simulink library "svm_lib"  (Simulink 8.6)
settings: Solver=VariableStepAuto  StartTime=0.0  StopTime=10.0  RelTol=1e-3
values from neighbouring files (symbols this model uses):
  My_3D = ([eye(6) -eye(6)])    [svm_buildLinearControllers.m]    (also in svm_setup.m = [-eye(6) eye(6)])
  turbulence2loadfactors = blkdiag(T_w2nx, T_w2nz)    [svm_buildLinearControllers.m]
  uavsim = loaded.uavsim    [svm_sandbox.m]
undefined symbols (not defined in the file or in its folder): dt, F, fflib_delay_c2d, Light, mask_p0_NED, mask_v0_NED, MIL, postracking, svm, uavsimblockset_cartesianToAngle
libraries: svm_lib x9, simulink_extras x8, aerolibtransform2 x3, formationFlyingBlockset x2, uavsimBlockset_Cularis_Aerandpropulsion x1, uavsimBlockset_ElectricPropulsion x1, aerolibwind2 x1, aerolibgravity2 x1, uavsimBlockset_VectorNorm x1, uavsimBlockset_UAV3DInterface x1
(part 3 of 3)

== system svm_lib/Standard Vehicle Model/Inner loop dynamics/Second order models ==
  u : Inport
  Bus Selector : BusSelector  OutputSignals=n
  Bus Object Bus Creator : BusCreator  Inputs=2  OutDataTypeStr=Bus: svm_bus_xi  mask(BUS OBJECT Bus Creator){busType=Bus: svm_bus_xi}
      mask prompts: busType "Bus Type"
      mask help:
      | Provides users the cabability to painlessly, instantly customize bus creators of output data type 'Bus:' by selecting the bus object type from a drop down menu dynamically populated by bus objects in the workspace.
      |
      | After pressing the "Apply Selection" button signal lines into the creator are populated and named with the elements in the chosen bus saving the user from having to recall and fill out signal line names.
      |
      | NOTE that when copying a Bus Object Bus Creator from your locked Library the link to the Library is automatically broken. This saves the user from having to Unlock Links To Library (From the Library menu.), Disable Link and finally Break Link (Both from the Model menu.) for every placed instance of the block.
      settings: AttributesFormatString=%<OutDataTypeStr>  CopyFcn=set_param(gcb, 'LinkStatus', 'none')
      mask TypeOptions busType: Bus: AHRS | Bus: Acceleration | Bus: Aero | Bus: Airdata | Bus: Airframe | Bus: Attitude | Bus: CMD | Bus: CMD_quadrotor | Bus: ControlInfoBus | Bus: Enginedata | Bus: Environment | Bus: FlightGearData | Bus: GCSUpstream | Bus: GNSSL1 | Bus: GNSSRTK | Bus: GPS | Bus: IMU | Bus: Kinematics | Bus: LandinggearInput | Bus: MotionTracker | Bus: Position | Bus: Radiodistance | Bus: RotationalAcceleration | Bus: RotationalVelocity | Bus: SensorBus | Bus: StateBus | Bus: Velocity | Bus: WindAngles | Bus: iUAScom | Bus: svm_bus_d_exo | Bus: svm_bus_u_scaled | Bus: svm_bus_x | Bus: svm_bus_xi
      mask Callback busType:
      | % Using variable names terminated with "_BOBC" to lessen the chances of
      | % collisions with existing workspace variables.
      | 
      | % Get the current block handle and mask handle.
      | handleCreator_BOBC = gcbh;
      | maskObj_BOBC       = Simulink.Mask.get(gcb);
      | 
      | % Get a list of variables in the workspace in order to search for the '1x1
      | % Bus' types.
      | wsVars_BOBC = whos;
      | 
      | % Reset the 'TypeOptions' bus list in case some '1x1 Bus' types have been
      | % deleted from or added to the workspace.
      | maskObj_BOBC.Parameters.TypeOptions = {'<empty>'};
      | 
      | % Reset the bus count.
      | busCount_BOBC = 0;
      | 
      | for index_BOBC = 1:length(wsVars_BOBC)
      | 
      |    % If the variable is a bus object...
      |    if strcmp(wsVars_BOBC(index_BOBC).class, 'Simulink.Bus')
      | 
      |       busCount_BOBC = busCount_BOBC + 1;
      | 
      |       % ... add it to the TypeOptions of the mask.
      |       maskObj_BOBC.Parameters.TypeOptions(busCount_BOBC) = ...
      |                                                            ...
      |                                  {['Bus: ', wsVars_BOBC(index_BOBC).name]};
      |    end
      | end
      | 
      | if busCount_BOBC == 0
      | 
      |    % If there are NO bus objects in the workspace then provide a warning
      |    % popup...
      |    warndlg('There are currently no bus objects in the workspace - you have no use for this block. Use a normal Bus Creator instead.')
      | 
      |    % ... and do nothing.
      | elseif ~strcmp(get_param(handleCreator_BOBC, 'OutDataTypeStr'), 'Inherit: auto')
      | 
      |    % If the currently selected bus data type ('OutDataTypeStr') is not
      |    % 'Inherit: auto' (i.e., if we are reopening the mask.) then get the
      |    % current 'OutDataTypeStr' and 'maskVal.' ('maskVal' is the selected
      |    % 'TypeOptions' list member.)
      |    outDatStr_BOBC = get_param(handleCreator_BOBC, 'OutDataTypeStr');
      |    maskVal_BOBC   = get_param(handleCreator_BOBC, 'MaskValues');
      | 
      |    if ~strcmp(outDatStr_BOBC, maskVal_BOBC{1})
      | 
      |       % Upon re-opening the mask if the default 'TypeOptions' list member
      |       % (The first one.) contained in 'maskVal' does not match the
      |       % currently selected bus data type ('OutDataTypeStr') then set the
      |       % 'TypeOptions' list member to the selected bus data type. (Cuts down
      |       % on confusion to have the displayed list member match the selected
      |       % bus data type rather than the first entry.)
      |       set_param(handleCreator_BOBC, 'MaskValues', {outDatStr_BOBC});
      |    end
      | end
      | 
      | % Clean up the workspace.
      | clear  handleCreator_BOBC  maskObj_BOBC     wsVars_BOBC ...
      |             busCount_BOBC    index_BOBC  outDatStr_BOBC ...
      |              maskVal_BOBC
      mask DialogControl applyMOCBSelection Prompt: Apply Selection
      mask DialogControl applyMOCBSelection Callback:
      | % Using variable names terminated with "_BOBC" to lessen the chances of
      | % collisions with existing workspace variables.
      | 
      | % Get the current block, current block handle and mask handle.
      | currentBlock_BOBC  = gcb;
      | handleCreator_BOBC = gcbh;
      | 
      | % Get the desired bus type...
      | desiredBusType_BOBC = get_param(handleCreator_BOBC, 'busType');
      | 
      | % ... and set the 'OutDataTypeStr' to it.
      | set_param(handleCreator_BOBC, 'OutDataTypeStr', desiredBusType_BOBC);
      | 
      | %% First delete any existing lines on the port.
      | % Get the line handles.
      | lh_BOBC = get_param(handleCreator_BOBC, 'LineHandles');
      | 
      | % If any lines exist (Non- -1 line handles.), delete them and start over.
      | if max(lh_BOBC.Inport > 0)
      | 
      |    for index_BOBC = 1:length(lh_BOBC.Inport)
      | 
      |       if lh_BOBC.Inport(index_BOBC) > 0
      | 
      |          delete_line(lh_BOBC.Inport(index_BOBC))
      |       end
      |    end
      | end
      | 
      | %% Then work on adding new lines.
      | 
      | % Get the block path for 'add_line' function.
      | blockPath_BOBC = get_param(handleCreator_BOBC, 'Parent');
      | 
      | % Get the newly selected bus type ('OutDataTypeStr')...
      | mocbBusType_BOBC = get_param(currentBlock_BOBC, 'OutDataTypeStr');
      | 
      | % ... and parse off "Bus: " so the string of the desired bus contained in
      | % 'OutDataTypeStr' matches the raw workspace bus names.
      | mocbBusType_BOBC = mocbBusType_BOBC(6:end);
      | 
      | % Then evaluate the string containing the workspace bus name which will
      | % load the desired bus parameters.
      | busParams_BOBC = eval(mocbBusType_BOBC);
      | 
      | % From the parameters grab the number of lines to add.
      | numLines_BOBC = length(busParams_BOBC.Elements);
      | 
      | % Set the number of inputs of the masked bus creator to the number of lines
      | % to add.
      | set_param(handleCreator_BOBC, 'Inputs', num2str(numLines_BOBC));
      | 
      | % Get (Inputs.) port handles so we can grab the positions of them.
      | ph_BOBC = get_param(handleCreator_BOBC, 'PortHandles');
      | 
      | for index_BOBC = 1:numLines_BOBC
      | 
      |    % Get the position of input port number 'index_BOBC'.
      |    portPos_BOBC = get_param(ph_BOBC.Inport(index_BOBC), 'Position');
      | 
      |    % Add a line from 50 pixels left of the port position to the port
      |    % position. (This must be done because it's the lines that get named,
      |    % not the port positions.)
      |    portLine_BOBC = add_line(blockPath_BOBC, [portPos_BOBC - [50 0]; portPos_BOBC]);
      | 
      |    % Rename the new line to the bus 'index_BOBC-st/nd/rd/th' element name.
      |    set_param(portLine_BOBC, 'Name', busParams_BOBC.Elements(index_BOBC).Name)
      | end
      | 
      | %% Cleanup the workspace.
      | clear    currentBlock_BOBC  handleCreator_BOBC      index_BOBC ...
      |        desiredBusType_BOBC             lh_BOBC  blockPath_BOBC ...
      |           mocbBusType_BOBC      busParams_BOBC   numLines_BOBC ...
      |                    ph_BOBC        portPos_BOBC   portLine_BOBC
  Demux1 : Demux  Outputs=3
  Mux : Mux  Inputs=3
  Transfer Fcn (with initial outputs) : simulink_extras/Additional Linear/Transfer Fcn (with initial outputs)  N=uavsim.cularis.linearModels.eulers.ss_nz_cl_sorder.num{1}  D=uavsim.cularis.linearModels.eulers.ss_nz_cl_sorder.den{1}  Y0=uavsim.svm.n0(3)  U0=uavsim.svm.n0(3)
  Transfer Fcn (with initial outputs)1 : simulink_extras/Additional Linear/Transfer Fcn (with initial outputs)  N=uavsim.cularis.linearModels.eulers.ss_ny_cl_sorder.num{1}  D=uavsim.cularis.linearModels.eulers.ss_ny_cl_sorder.den{1}  Y0=uavsim.svm.n0(2)  U0=uavsim.svm.n0(2)
  Transfer Fcn (with initial outputs)2 : simulink_extras/Additional Linear/Transfer Fcn (with initial outputs)  N=uavsim.cularis.linearModels.eulers.ss_nx_cl_sorder.num{1}  D=uavsim.cularis.linearModels.eulers.ss_nx_cl_sorder.den{1}  Y0=uavsim.svm.n0(1)  U0=uavsim.svm.n0(1)
  not used : Constant  Value=zeros(3,1)
  x_i : Outport
  wires:
  Transfer Fcn (with initial outputs)/1 -> Mux/3
  Demux1/3 -> Transfer Fcn (with initial outputs)/1
  Demux1/2 -> Transfer Fcn (with initial outputs)1/1
  Demux1/1 -> Transfer Fcn (with initial outputs)2/1
  Transfer Fcn (with initial outputs)2/1 -> Mux/1
  Transfer Fcn (with initial outputs)1/1 -> Mux/2
  Bus Object Bus Creator/1 -> x_i/1
  u/1 -> Bus Selector/1
  Bus Selector/1 -> Demux1/1  "<n>"
  Mux/1 -> Bus Object Bus Creator/1  "n"
  not used/1 -> Bus Object Bus Creator/2  "ndot"

== system svm_lib/Standard Vehicle Model/Inner loop dynamics/Timescale separation ==
  u : Inport
  Bus Selector : BusSelector  OutputSignals=n
  Bus Object Bus Creator : BusCreator  Inputs=2  OutDataTypeStr=Bus: svm_bus_xi  mask(BUS OBJECT Bus Creator){busType=Bus: svm_bus_xi}
      mask prompts: busType "Bus Type"
      mask help:
      | Provides users the cabability to painlessly, instantly customize bus creators of output data type 'Bus:' by selecting the bus object type from a drop down menu dynamically populated by bus objects in the workspace.
      |
      | After pressing the "Apply Selection" button signal lines into the creator are populated and named with the elements in the chosen bus saving the user from having to recall and fill out signal line names.
      |
      | NOTE that when copying a Bus Object Bus Creator from your locked Library the link to the Library is automatically broken. This saves the user from having to Unlock Links To Library (From the Library menu.), Disable Link and finally Break Link (Both from the Model menu.) for every placed instance of the block.
      settings: AttributesFormatString=%<OutDataTypeStr>  CopyFcn=set_param(gcb, 'LinkStatus', 'none')
      mask TypeOptions busType: Bus: Acceleration | Bus: Aero | Bus: Airframe | Bus: Attitude | Bus: CMD | Bus: Environment | Bus: FlightGearData | Bus: Kinematics | Bus: Position | Bus: RotationalAcceleration | Bus: RotationalVelocity | Bus: Velocity | Bus: svm_bus_d_exo | Bus: svm_bus_u | Bus: svm_bus_x | Bus: svm_bus_xi
      mask Callback busType:
      | % Using variable names terminated with "_BOBC" to lessen the chances of
      | % collisions with existing workspace variables.
      | 
      | % Get the current block handle and mask handle.
      | handleCreator_BOBC = gcbh;
      | maskObj_BOBC       = Simulink.Mask.get(gcb);
      | 
      | % Get a list of variables in the workspace in order to search for the '1x1
      | % Bus' types.
      | wsVars_BOBC = whos;
      | 
      | % Reset the 'TypeOptions' bus list in case some '1x1 Bus' types have been
      | % deleted from or added to the workspace.
      | maskObj_BOBC.Parameters.TypeOptions = {'<empty>'};
      | 
      | % Reset the bus count.
      | busCount_BOBC = 0;
      | 
      | for index_BOBC = 1:length(wsVars_BOBC)
      | 
      |    % If the variable is a bus object...
      |    if strcmp(wsVars_BOBC(index_BOBC).class, 'Simulink.Bus')
      | 
      |       busCount_BOBC = busCount_BOBC + 1;
      | 
      |       % ... add it to the TypeOptions of the mask.
      |       maskObj_BOBC.Parameters.TypeOptions(busCount_BOBC) = ...
      |                                                            ...
      |                                  {['Bus: ', wsVars_BOBC(index_BOBC).name]};
      |    end
      | end
      | 
      | if busCount_BOBC == 0
      | 
      |    % If there are NO bus objects in the workspace then provide a warning
      |    % popup...
      |    warndlg('There are currently no bus objects in the workspace - you have no use for this block. Use a normal Bus Creator instead.')
      | 
      |    % ... and do nothing.
      | elseif ~strcmp(get_param(handleCreator_BOBC, 'OutDataTypeStr'), 'Inherit: auto')
      | 
      |    % If the currently selected bus data type ('OutDataTypeStr') is not
      |    % 'Inherit: auto' (i.e., if we are reopening the mask.) then get the
      |    % current 'OutDataTypeStr' and 'maskVal.' ('maskVal' is the selected
      |    % 'TypeOptions' list member.)
      |    outDatStr_BOBC = get_param(handleCreator_BOBC, 'OutDataTypeStr');
      |    maskVal_BOBC   = get_param(handleCreator_BOBC, 'MaskValues');
      | 
      |    if ~strcmp(outDatStr_BOBC, maskVal_BOBC{1})
      | 
      |       % Upon re-opening the mask if the default 'TypeOptions' list member
      |       % (The first one.) contained in 'maskVal' does not match the
      |       % currently selected bus data type ('OutDataTypeStr') then set the
      |       % 'TypeOptions' list member to the selected bus data type. (Cuts down
      |       % on confusion to have the displayed list member match the selected
      |       % bus data type rather than the first entry.)
      |       set_param(handleCreator_BOBC, 'MaskValues', {outDatStr_BOBC});
      |    end
      | end
      | 
      | % Clean up the workspace.
      | clear  handleCreator_BOBC  maskObj_BOBC     wsVars_BOBC ...
      |             busCount_BOBC    index_BOBC  outDatStr_BOBC ...
      |              maskVal_BOBC
      mask DialogControl applyMOCBSelection Prompt: Apply Selection
      mask DialogControl applyMOCBSelection Callback:
      | % Using variable names terminated with "_BOBC" to lessen the chances of
      | % collisions with existing workspace variables.
      | 
      | % Get the current block, current block handle and mask handle.
      | currentBlock_BOBC  = gcb;
      | handleCreator_BOBC = gcbh;
      | 
      | % Get the desired bus type...
      | desiredBusType_BOBC = get_param(handleCreator_BOBC, 'busType');
      | 
      | % ... and set the 'OutDataTypeStr' to it.
      | set_param(handleCreator_BOBC, 'OutDataTypeStr', desiredBusType_BOBC);
      | 
      | %% First delete any existing lines on the port.
      | % Get the line handles.
      | lh_BOBC = get_param(handleCreator_BOBC, 'LineHandles');
      | 
      | % If any lines exist (Non- -1 line handles.), delete them and start over.
      | if max(lh_BOBC.Inport > 0)
      | 
      |    for index_BOBC = 1:length(lh_BOBC.Inport)
      | 
      |       if lh_BOBC.Inport(index_BOBC) > 0
      | 
      |          delete_line(lh_BOBC.Inport(index_BOBC))
      |       end
      |    end
      | end
      | 
      | %% Then work on adding new lines.
      | 
      | % Get the block path for 'add_line' function.
      | blockPath_BOBC = get_param(handleCreator_BOBC, 'Parent');
      | 
      | % Get the newly selected bus type ('OutDataTypeStr')...
      | mocbBusType_BOBC = get_param(currentBlock_BOBC, 'OutDataTypeStr');
      | 
      | % ... and parse off "Bus: " so the string of the desired bus contained in
      | % 'OutDataTypeStr' matches the raw workspace bus names.
      | mocbBusType_BOBC = mocbBusType_BOBC(6:end);
      | 
      | % Then evaluate the string containing the workspace bus name which will
      | % load the desired bus parameters.
      | busParams_BOBC = eval(mocbBusType_BOBC);
      | 
      | % From the parameters grab the number of lines to add.
      | numLines_BOBC = length(busParams_BOBC.Elements);
      | 
      | % Set the number of inputs of the masked bus creator to the number of lines
      | % to add.
      | set_param(handleCreator_BOBC, 'Inputs', num2str(numLines_BOBC));
      | 
      | % Get (Inputs.) port handles so we can grab the positions of them.
      | ph_BOBC = get_param(handleCreator_BOBC, 'PortHandles');
      | 
      | for index_BOBC = 1:numLines_BOBC
      | 
      |    % Get the position of input port number 'index_BOBC'.
      |    portPos_BOBC = get_param(ph_BOBC.Inport(index_BOBC), 'Position');
      | 
      |    % Add a line from 50 pixels left of the port position to the port
      |    % position. (This must be done because it's the lines that get named,
      |    % not the port positions.)
      |    portLine_BOBC = add_line(blockPath_BOBC, [portPos_BOBC - [50 0]; portPos_BOBC]);
      | 
      |    % Rename the new line to the bus 'index_BOBC-st/nd/rd/th' element name.
      |    set_param(portLine_BOBC, 'Name', busParams_BOBC.Elements(index_BOBC).Name)
      | end
      | 
      | %% Cleanup the workspace.
      | clear    currentBlock_BOBC  handleCreator_BOBC      index_BOBC ...
      |        desiredBusType_BOBC             lh_BOBC  blockPath_BOBC ...
      |           mocbBusType_BOBC      busParams_BOBC   numLines_BOBC ...
      |                    ph_BOBC        portPos_BOBC   portLine_BOBC
  Constant : Constant  Value=[0 0 0]'
  x_i : Outport
  wires:
  u/1 -> Bus Selector/1
  Bus Object Bus Creator/1 -> x_i/1
  Bus Selector/1 -> Bus Object Bus Creator/1  "<n>"
  Constant/1 -> Bus Object Bus Creator/2  "ndot"

== matlab function SMC/STSMC z/MATLAB Function ==
  data: u1 output double; dp input double; dv input double; par input double; w output double; sigma output double; u input double
function [u1, w, sigma ] = fcn(dp, dv, par, u)
%#codegen
u1 = 0;
sigma = 0;
persistent lastsample;
if isempty(lastsample)
    lastsample.sigma = 0;
end
sigma = par.supertwist_lambda1*dp + dv;
% Discrete approximation of sigmaDot:
sigmaDot = sigma - lastsample.sigma;
lastsample.sigma = sigma;

u1 = - par.supertwist_alpha * sqrt(norm(sigma)) * sign(sigma);
if abs(u) > par.supertwist_umax
    w = - u;
else
    w = -par.supertwist_r1*sign(sigma) - par.supertwist_r2*sign(sigmaDot);
end

== matlab function SMC/STSMC x/MATLAB Function ==
  data: u1 output double; dp input double; dv input double; par input double; w output double; sigma output double; u input double
function [u1, w, sigma ] = fcn(dp, dv, par, u)
%#codegen
u1 = 0;
sigma = 0;
persistent lastsample;
if isempty(lastsample)
    lastsample.sigma = 0;
end
sigma = par.supertwist_lambda1*dp + dv;
% Discrete approximation of sigmaDot:
sigmaDot = sigma - lastsample.sigma;
lastsample.sigma = sigma;

u1 = - par.supertwist_alpha * sqrt(norm(sigma)) * sign(sigma);
if abs(u) > par.supertwist_umax
    w = - u;
else
    w = -par.supertwist_r1*sign(sigma) - par.supertwist_r2*sign(sigmaDot);
end

bp = 0;
end

== matlab function SMC/STSMC y/MATLAB Function ==
  data: u1 output double; dp input double; dv input double; par input double; w output double; sigma output double; u input double
function [u1, w, sigma ] = fcn(dp, dv, par, u)
%#codegen
u1 = 0;
sigma = 0;
persistent lastsample;
if isempty(lastsample)
    lastsample.sigma = 0;
end
sigma = par.supertwist_lambda1*dp + dv;
% Discrete approximation of sigmaDot:
sigmaDot = sigma - lastsample.sigma;
lastsample.sigma = sigma;

u1 = - par.supertwist_alpha * sqrt(norm(sigma)) * sign(sigma);
if abs(u) > par.supertwist_umax
    w = - u;
else
    w = -par.supertwist_r1*sign(sigma) - par.supertwist_r2*sign(sigmaDot);
end

== matlab function SMC/STSMC z/MATLAB Function1 ==
  data: x input double; y output double; sigma output double
function [y, sigma] = fcn(x)
coder.extrinsic('evalin')
G = zeros(1,2);
A = zeros(2,2);
B = zeros(2,1);
dt = 0;
G = evalin('base', 'G');
A = evalin('base', 'A');
B = evalin('base', 'B');
dt = 15*evalin('base', 'dt');

ueq = -(G*B)^-1*G*A*x;

sigma = G*x;
% Explicit:
udisc_expl = -sign(sigma);
% Implicit:
udisc_impl = 0;
if abs(sigma) <= dt
    udisc_impl =  -sigma/dt;
elseif sigma > dt
    udisc_impl = -1;
elseif sigma < -dt
    udisc_impl = 1;
end

y = 0;
y = ueq +  1*udisc_impl;
end

== matlab function implicit euler ==
  data: x input double; u output double; sigma output double; tsim input double
function [u, sigma] = fcn(x, tsim)
coder.extrinsic('evalin');
coder.extrinsic('sandbox_extrinsic_zeroorder');
% G = zeros(1,2);
dt = 0;
a = zeros(1);
b = zeros(1);
% G = evalin('base', 'G');
a = evalin('base', 'a');
b = evalin('base', 'b');
dt = evalin('base', 'postracking.T');
G = [6 4];
%
% ueq = -(G*B)^-1*G*A*x;
%
sigma = G*x;

% Explicit:
udisc_expl = -sign(sigma);

% Implicit:
udisc_impl = 0;
if abs(sigma) <= dt
    udisc_impl =  - sigma/dt;
elseif sigma > dt
    udisc_impl = -1;
elseif sigma < -dt
    udisc_impl = 1;
end

u = 0;
u =  -1*udisc_expl;

if abs(sigma) <= 1e-1
 %   tic;
   %u = sandbox_extrinsic_zeroorder(x, G, dt, a, b);
%   toc
end

end

== matlab function CSTSMC/MATLAB Function ==
  data: u1 output double; dp input double; dv input double; da input double; w output double; sigma output double; u input double
function [u1, w, sigma ] = cstscm(dp, dv, da, u)
coder.extrinsic('cstscm_extrinsic');
coder.extrinsic('angle2dcm');
coder.extrinsic('evalin');

u1 = zeros(3,1);
w = zeros(3,1);
sigma = zeros(3,1);
N = zeros(3,1);

%[u1, w, sigma] = cstscm_extrinsic(dp, dv, da, u);

u1 = zeros(3,1);
w = zeros(3,1);
persistent lastsample;
if isempty(lastsample)
    lastsample.sigma = zeros(3,1);
    N = evalin('base', 'uavsim.svm.usat.n_c.upper')';
end

lp = [6 6 6];
lv = [4 4 4];
G = [diag(lp) diag(lv)];
sigma = G * [dp; dv];
lastsample.sigma = sigma;

% Compute controller in compliance with ACA article:
% Known disturbances:
B = [zeros(3); eye(3)];
phi_k = [dv;
    [0; 0; 9.81]];
phi_k_apostroph = G*phi_k;
upre = (1/9.81)*(G*B)^(-1)*phi_k_apostroph;

% Upper bounds on unknown disturbances:
Aw = [1 1 0.46 + 0.0083]';
%max load factors:
R_be = eye(3);
R_be = eye(3); %angle2dcm(0,0,0);
R_eb = R_be';
nc0 = R_be * [0 0 -1]';
U =  R_eb * 9.81 * (N - nc0);
apre_max = U;
phiu_max = Aw + apre_max;
phiuapostroph_max = G*B*phiu_max;
L = phiuapostroph_max;

% Run three SISO controllers:
for k=1:3
    alpha = 1.5*sqrt(L(k));
    beta = 1.1*L(k);
    u1(k) =   alpha * sqrt(norm(sigma(k))) * sign(sigma(k)) + upre(k);
    %if abs(u) > par(6)
    %    w =  - u;
    %else
    w(k) =  beta*sign(sigma(k));
    %end
end
end

== matlab function SMC-directforce/implicit euler ==
  data: x input double; u output double; sigma output double; tsim input double
function [u, sigma] = fcn(x, tsim)
coder.extrinsic('evalin');
coder.extrinsic('sandbox_extrinsic_zeroorder');
% G = zeros(1,2);
dt = 0;
a = zeros(1);
b = zeros(1);
% G = evalin('base', 'G');
a = evalin('base', 'a');
b = evalin('base', 'b');
dt = evalin('base', 'postracking.T');
G = [6 4];
%
% ueq = -(G*B)^-1*G*A*x;
%
sigma = G*x;

% Explicit:
udisc_expl = -sign(sigma);

% Implicit:
udisc_impl = 0;
if abs(sigma) <= dt
    udisc_impl =  - sigma/dt;
elseif sigma > dt
    udisc_impl = -1;
elseif sigma < -dt
    udisc_impl = 1;
end

u = 0;
u =  -1*udisc_expl;

if abs(sigma) <= 1e-1
 %   tic;
   %u = sandbox_extrinsic_zeroorder(x, G, dt, a, b);
%   toc
end

end

== matlab function PDSMC/MATLAB Function ==
  data: nc output double; dp input double; dv input double; da input double; sigma output double; dbport output double; tsim input double
function [nc, sigma, dbport ] = dsmc(dp, dv, da, tsim)
coder.extrinsic('dsmc_extrinsic');

nc = zeros(3,1);
sigma = zeros(3,1);
dbport = zeros(1,1);

[nc, sigma, dbport] = dsmc_extrinsic(dp, dv, da, tsim);

end
